simulink model "model6"  (R2019b)
settings: Solver=VariableStepAuto  StartTime=0.0  StopTime=10.0  RelTol=1e-3
libraries: simulink x1
settings Model: Creator=surtweig  LastModifiedBy=surtweig

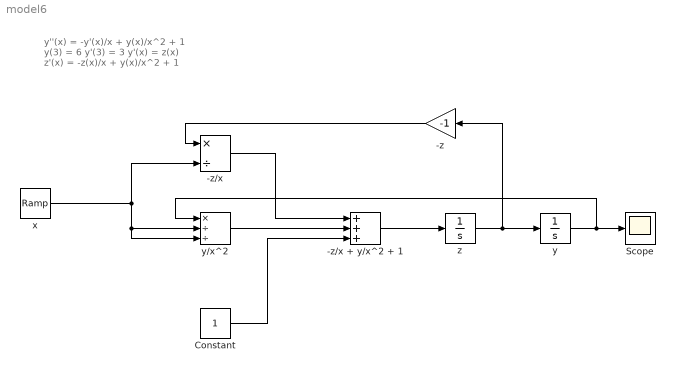
== system model6 ==
  note: y''(x) = -y'(x)/x + y(x)/x^2 + 1
      | y(3) = 6
      | y'(3) = 3
      |
      | y'(x) = z(x)
      | z'(x) = -z(x)/x + y(x)/x^2 + 1
  -z : Gain  Gain=-1
  -z/x : Product  Inputs=*/
  -z/x + y/x^2 + 1 : Sum  Inputs=+++
  Constant : Constant
  Scope : Scope
  x : simulink/Sources/Ramp  slope=1  start=0  InitialOutput=3
  y : Integrator  InitialCondition=6
  y/x^2 : Product  Inputs=*//
  z : Integrator  InitialCondition=3
  wires:
  z/1 -> -z/1, y/1
  y/1 -> y/x^2/1, Scope/1
  -z/x + y/x^2 + 1/1 -> z/1
  Constant/1 -> -z/x + y/x^2 + 1/3
  y/x^2/1 -> -z/x + y/x^2 + 1/2
  -z/x/1 -> -z/x + y/x^2 + 1/1
  -z/1 -> -z/x/1
  x/1 -> y/x^2/2, y/x^2/3, -z/x/2
